simulink model "lab2_block"  (R2017b)
settings: Solver=VariableStepAuto  StartTime=0.0  StopTime=10  RelTol=1e-3
settings Model: Creator=user  LastModifiedBy=HONOR
settings SolverCC: AutoInsertRateTranBlk=on
settings DataIOCC: LimitDataPoints=on  SaveOutput=off  SignalLogging=off  SaveTime=off
settings OptimizationCC: LifeSpan=inf
settings DebuggingCC: AlgebraicLoopMsg=error  SingleTaskRateTransMsg=error  AllowSymbolicDim=off  SFUnexpectedBacktrackingDiag=warning  SFNoUnconditionalDefaultTransitionDiag=warning  SFExecutionAtInitializationDiag=none
settings CodeAppCC: StateflowObjectComments=on
settings GRTTargetCC: TargetLangStandard=C89/C90 (ANSI)  GeneratePreprocessorConditionals=Disable all
settings ConfigComp: CovMetricSettings=dw  CovHtmlReporting=on  CovSaveCumulativeToWorkspaceVar=on  CovSaveSingleToWorkspaceVar=on  CovExternalEMLEnable=off

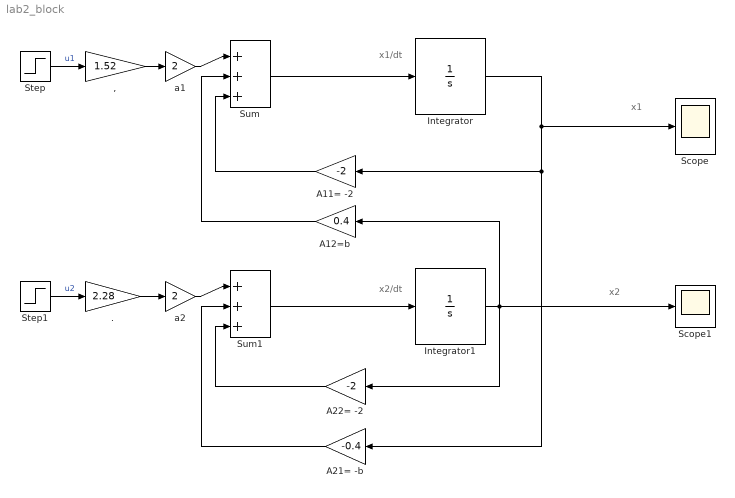
== system lab2_block ==
  note: x2
  note: x2/dt
  note: x1
  note: x1/dt
  , : Gain  Gain=1.52
  . : Gain  Gain=2.28
  A11= -2 : Gain  Gain=-2
  A12=b : Gain  Gain=0.4
  "A21= -b " : Gain  Gain=-0.4
  A22= -2 : Gain  Gain=-2
  Integrator : Integrator
  Integrator1 : Integrator
  Scope : Scope
  Scope1 : Scope
  Step : Step  Time=0  SampleTime=0
  Step1 : Step  Time=0  SampleTime=0
  Sum : Sum  Inputs=|+++
  Sum1 : Sum  Inputs=|+++
  a1 : Gain  Gain=2
  a2 : Gain  Gain=2
  wires:
  Sum/1 -> Integrator/1
  Sum1/1 -> Integrator1/1
  Integrator/1 -> "A21= -b "/1, A11= -2/1, Scope/1
  A11= -2/1 -> Sum/3
  Integrator1/1 -> Scope1/1, A22= -2/1, A12=b/1
  A12=b/1 -> Sum/2
  A22= -2/1 -> Sum1/3
  "A21= -b "/1 -> Sum1/2
  a2/1 -> Sum1/1
  Step/1 -> ,/1  "u1"
  a1/1 -> Sum/1
  ,/1 -> a1/1
  Step1/1 -> ./1  "u2"
  ./1 -> a2/1
